simulink model "sl_robot"  (R2014a)
settings: Solver=ode45  StartTime=0.0  StopTime=30  FixedStep=0.01  RelTol=1e-3
PreLoadFcn:
  | puma560
  | p560 = nofriction(p560);
values from neighbouring files (symbols this model uses):
  complex_leg = SerialLink(complex_leg_links, 'name', 'complex_leg', 'offset', complex_leg_offsets)    [project.m]
undefined symbols (not defined in the file or in its folder): W_adapt_matrix
libraries: roblocks x3
settings Model: ExtModeTrigMode=oneshot  ExtModeArmWhenConnect=off  Creator=pic  LastModifiedBy=pavelmironchyk
settings DataIOCC: LimitDataPoints=off  SignalLoggingSaveFormat=ModelDataLogs  ReturnWorkspaceOutputs=on
settings OptimizationCC: BlockReduction=off  BooleanDataType=off  ExpressionDepthLimit=2147483647  InitFltsAndDblsToZero=on
settings DebuggingCC: SaveWithParameterizedLinksMsg=none  UnderspecifiedInitializationDetection=Classic  SignalResolutionControl=TryResolveAllWithWarning  SolverPrmCheckMsg=none  MultiTaskDSMMsg=warning  MultiTaskCondExecSysMsg=none  FcnCallInpInsideContextMsg=UseLocalSettings  StateNameClashWarn=warning
settings HardwareCC: TargetUnknown=on
settings RTWCC: IncludeERTFirstTime=on
settings GRTTargetCC: ModelReferenceCompliant=off  CompOptLevelCompliant=off  CombineOutputUpdateFcns=off  MatFileLogging=off  GRTInterface=on

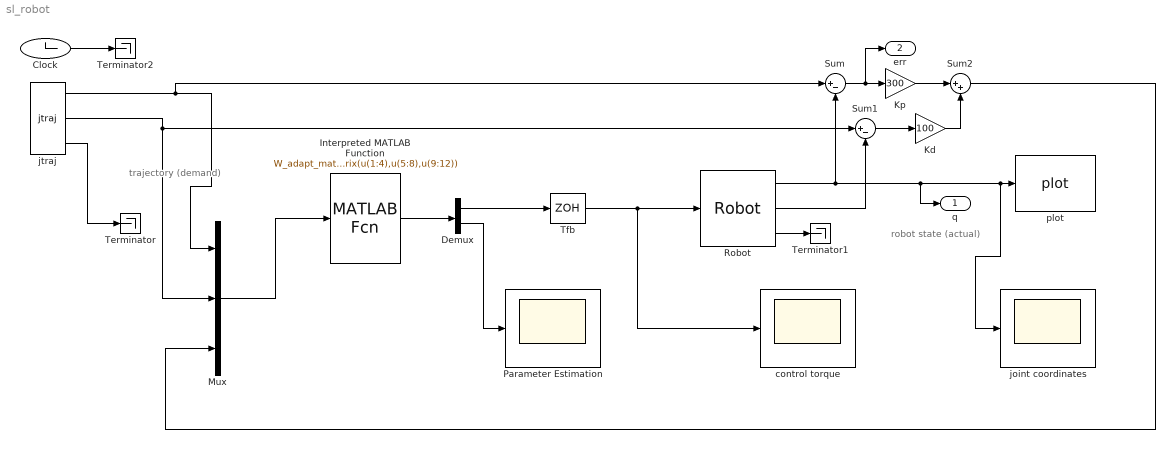
== system sl_robot ==
  note: trajectory
      | (demand)
  note: robot state
      | (actual)
  Clock : Clock
  Demux : Demux  Outputs=2
  Interpreted MATLAB Function : MATLABFcn  MATLABFcn=W_adapt_matrix(u(1:4),u(5:8),u(9:12))  OutputDimensions=9  OutputSignalType=real
  Kd : Gain  Gain=100  SaturateOnIntegerOverflow=on  OutDataTypeStr=Inherit: Same as input  ParamDataTypeStr=Inherit: Same as input
  Kp : Gain  Gain=300  SaturateOnIntegerOverflow=on  OutDataTypeStr=Inherit: Same as input  ParamDataTypeStr=Inherit: Same as input
  Mux : Mux  Inputs=3
  Parameter Estimation : Scope
      settings: TimeRange=0.14  YMin=-8.13152e-20  YMax=0.0015  SaveName=ScopeData2
  Robot : roblocks/Dynamics/Robot  robot=complex_leg.nofriction()  q0=[0 0 0 0]
  Sum : Sum  Inputs=|+-  SaturateOnIntegerOverflow=on  InputSameDT=on  OutDataTypeStr=Inherit: Same as first input
  Sum1 : Sum  Inputs=|+-  SaturateOnIntegerOverflow=on  InputSameDT=on  OutDataTypeStr=Inherit: Same as first input
  Sum2 : Sum  Inputs=|++  SaturateOnIntegerOverflow=on  InputSameDT=on  OutDataTypeStr=Inherit: Same as first input
  Terminator : Terminator
  Terminator1 : Terminator
  Terminator2 : Terminator
  Tfb : ZeroOrderHold  SampleTime=0.01
  "control torque " : Scope
      settings: TimeRange=10  YMin=-0.015  YMax=0.015
  joint coordinates : Scope
      settings: TimeRange=10  YMin=-0.375  YMax=0.2
  jtraj : roblocks/Trajectory/jtraj  q0=[0 0 0 0]  qf=[pi/3 -pi/6 pi/4 pi/4 ]  tmax=30  ts=0.02
  plot : roblocks/Robot Graphics/plot  robot=complex_leg  fps=25  holdplot=off
  q : Outport
  err : Outport  Port=2
  wires:
  Sum/1 -> Kp/1, err/1
  Kp/1 -> Sum2/1
  Robot/1 -> joint coordinates/1, plot/1, q/1, Sum/2
  Robot/2 -> Sum1/2
  Sum2/1 -> Mux/3
  jtraj/1 -> Sum/1, Mux/1
  jtraj/2 -> Sum1/1, Mux/2
  Sum1/1 -> Kd/1
  Kd/1 -> Sum2/2
  jtraj/3 -> Terminator/1
  Robot/3 -> Terminator1/1
  Tfb/1 -> "control torque "/1, Robot/1
  Clock/1 -> Terminator2/1
  Mux/1 -> Interpreted MATLAB Function/1
  Interpreted MATLAB Function/1 -> Demux/1
  Demux/1 -> Tfb/1
  Demux/2 -> Parameter Estimation/1
